simulink model "LMS_ANC"  (R2023a)
settings: Solver=VariableStepAuto  StartTime=0.0  StopTime=10  RelTol=1e-3
model workspace (MAT data in the model file):
  w = [0.5 0.5]
libraries: dspsnks4 x1, dspadpt3 x1, dspsrcs4 x1
settings Model: Creator=logan  LastModifiedBy=logan
settings DebuggingCC: ParameterPrecisionLossMsg=none

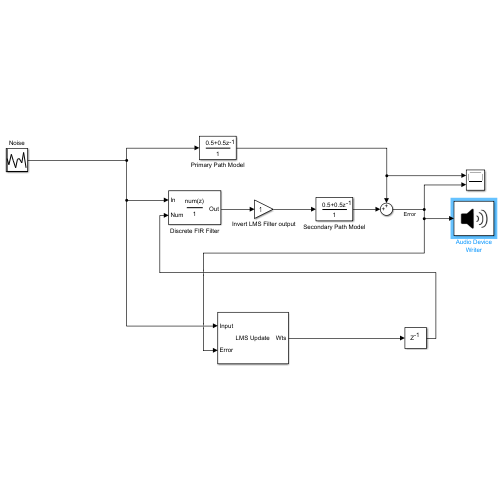
[thumbnail: Simulink's stored preview of the top-level diagram]
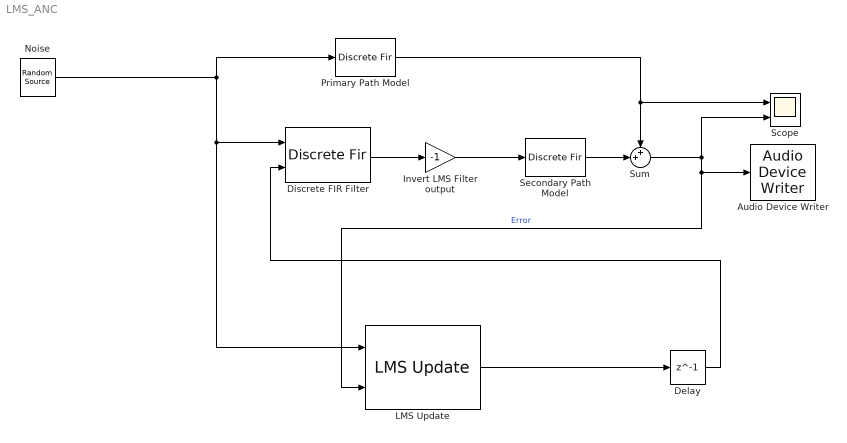
== system LMS_ANC ==
  Audio Device Writer : dspsnks4/Audio Device Writer  Driver=DirectSound  Device=Default  InheritSampleRate=on  SampleRate=44100  BitDepth=16-bit integer  BufferSize=4096  NumBuffers=10  DefaultOutputChannelMapping=on  OutputChannelMapping=1:2  OutputNumUnderrunSamples=off  DriverIdx=1  DeviceWarnFlag=''
  Delay : Delay  DelayLength=1
  Discrete FIR Filter : DiscreteFir  CoefSource=Input port
      settings: InputPortMap=u0,u1
  Invert LMS Filter output : Gain  Gain=-1
  LMS Update : dspadpt3/LMS Update  Method=LMS  Length=32  NumFilters=1  StepSizeSource=Property  StepSize=0.01  LeakageFactor=1.0  InitialConditions=0  AdaptiveFilterMode=Tapped delay-line FIR filter  EnableAdaptInput=off  EnableResetInput=off  SimulateUsing=Code generation
  Noise : dspsrcs4/Random Source  SrcType=Gaussian  NormMethod=Sum of uniform values  CltLength=5  MinVal=-1  MaxVal=1  MeanVal=0  VarVal=1  RepMode=Specify seed  rawSeed=[23341]  IsInherit=off  SampMode=Discrete  SampTime=1/8000  SampFrame=1  DataType=Single  OutComplex=Real  OutputFrames=off
  Primary Path Model : DiscreteFir
  Scope : Scope  NumInputPorts=2
  Secondary Path Model : DiscreteFir
  Sum : Sum  Inputs=++|
  wires:
  Sum/1 -> Scope/2, LMS Update/2, Audio Device Writer/1  "Error"
  LMS Update/1 -> Delay/1
  Discrete FIR Filter/1 -> Invert LMS Filter output/1
  Invert LMS Filter output/1 -> Secondary Path Model/1
  Delay/1 -> Discrete FIR Filter/2
  Primary Path Model/1 -> Sum/1, Scope/1
  Secondary Path Model/1 -> Sum/2
  Noise/1 -> LMS Update/1, Discrete FIR Filter/1, Primary Path Model/1
